simulink model "FuzzyLogicRobot_rev3"  (R2014a)
settings: Solver=ode45  SolverMode=SingleTasking  StartTime=0  StopTime=4.6  MaxStep=0.05  RelTol=1e-3  AbsTol=1e-6
libraries: simulink x3, fuzblock x1
CloseFcn:
  | AnimFigH = findobj(0,'Name', 'Tank Demo'); close(AnimFigH)
Description:
  | Control difuso de un robot móvil del tipo diferencial
settings Model: NumberOfSteps=10  LastModifiedBy=fravega
settings DataIOCC: LimitDataPoints=off  SignalLoggingSaveFormat=ModelDataLogs  SaveOutput=off  SaveTime=off
settings OptimizationCC: BlockReduction=off  BooleanDataType=off  ExpressionDepthLimit=2147483647  InitFltsAndDblsToZero=on
settings DebuggingCC: SaveWithParameterizedLinksMsg=none  UnderspecifiedInitializationDetection=Classic  SignalResolutionControl=TryResolveAllWithWarning  SolverPrmCheckMsg=none  MultiTaskDSMMsg=warning  MultiTaskCondExecSysMsg=none  FcnCallInpInsideContextMsg=UseLocalSettings  StateNameClashWarn=warning
settings HardwareCC: TargetLongLongMode=on  TargetEndianess=LittleEndian  TargetHWDeviceType=MATLAB Host  ProdEqTarget=off
settings RTWCC: GenerateMakefile=off  TemplateMakefile=grt_unix.tmf  IncludeERTFirstTime=on
settings GRTTargetCC: TargetFcnLib=ansi_tfl_tmw.mat  CombineOutputUpdateFcns=off  GRTInterface=on

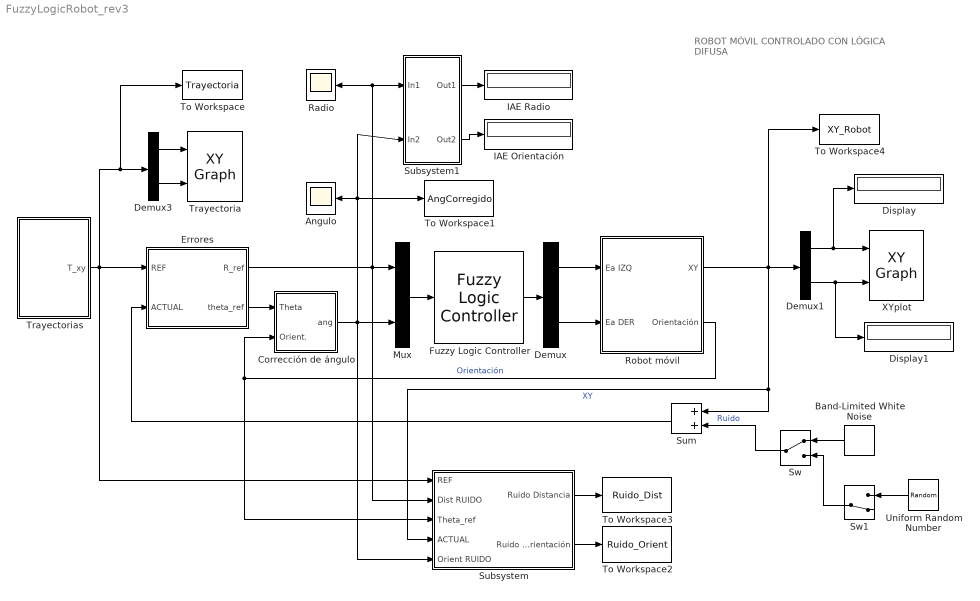
== system FuzzyLogicRobot_rev3 ==
  note: ROBOT MÓVIL CONTROLADO
      |  CON LÓGICA DIFUSA
  Angulo : Scope
      settings: TimeRange=5  YMin=-10  YMax=50  SaveName=ScopeData9
  Band-Limited White Noise : simulink/Sources/Band-Limited White Noise  Cov=[0.003]  Ts=0.1  seed=[23341]
  Corrección de ángulo : Subsystem
  Demux : Demux  Outputs=2
  Demux1 : Demux  Outputs=2
  Demux3 : Demux  Outputs=2
  Display : Display
  Display1 : Display
  Errores : Subsystem
  Fuzzy Logic Controller : fuzblock/Fuzzy Logic  Controller  fis='MRFL_rev33.fis'
  "IAE Orientación " : Display
  IAE Radio : Display
  Mux : Mux  Inputs=2
  Radio : Scope
      settings: TimeRange=5  YMin=0  SaveName=ScopeData10
  Robot móvil : Subsystem
      mask help:
      | Robot móvil del tipo Diferencial
      |
      | Entradas: Tensión de armadura de los motores de DC
      | Salidas: Posición en el plano (XY) y orientación
      mask Display: image('DDR.jpg')
  Subsystem : Subsystem
  Subsystem1 : Subsystem
  Sum : Sum
  Sw : ManualSwitch
  Sw1 : ManualSwitch  CurrentSetting=0
  To Workspace : ToWorkspace  VariableName=Trayectoria  SaveFormat=Timeseries  SampleTime=-1
  To Workspace1 : ToWorkspace  VariableName=AngCorregido  SaveFormat=Timeseries  SampleTime=-1
  To Workspace2 : ToWorkspace  VariableName=Ruido_Orient  SaveFormat=Timeseries  SampleTime=-1
  To Workspace3 : ToWorkspace  VariableName=Ruido_Dist  SaveFormat=Timeseries  SampleTime=-1
  To Workspace4 : ToWorkspace  VariableName=XY_Robot  SaveFormat=Timeseries  SampleTime=-1
  "Trayectoria " : simulink/Sinks/XY Graph  xmin=-4  xmax=4  ymin=-4  ymax=4  st=-1
  Trayectorias : Subsystem
  Uniform Random Number : UniformRandomNumber  SampleTime=0.1
  XYplot : simulink/Sinks/XY Graph  xmin=-4  xmax=4  ymin=-4  ymax=4  st=-1
  wires:
  Mux/1 -> Fuzzy Logic Controller/1
  Errores/2(theta_ref) -> Corrección de ángulo/1(Theta)
  Corrección de ángulo/1(ang) -> Angulo/1, To Workspace1/1, Subsystem1/2(In2), Subsystem/5(Orient RUIDO), Mux/2
  Trayectorias/1(T_xy) -> Subsystem/1(REF), Errores/1(REF), To Workspace/1, Demux3/1
  Robot móvil/1(XY) -> To Workspace4/1, Demux1/1, Sum/1, Subsystem/4(ACTUAL)  "XY"
  Errores/1(R_ref) -> Radio/1, Subsystem1/1(In1), Subsystem/2(Dist RUIDO), Mux/1
  Fuzzy Logic Controller/1 -> Demux/1
  Band-Limited White Noise/1 -> Sw/1
  Sw/1 -> Sum/2  "Ruido"
  Robot móvil/2(Orientación) -> Corrección de ángulo/2(Orient.), Subsystem/3(Theta_ref)  "Orientación"
  Sw1/1 -> Sw/2
  Uniform Random Number/1 -> Sw1/1
  Demux3/1 -> "Trayectoria "/1
  Demux3/2 -> "Trayectoria "/2
  Sum/1 -> Errores/2(ACTUAL)
  Demux/2 -> Robot móvil/2(Ea DER)
  Demux/1 -> Robot móvil/1(Ea IZQ)
  Demux1/1 -> XYplot/1, Display/1
  Demux1/2 -> Display1/1, XYplot/2
  Subsystem1/1(Out1) -> IAE Radio/1
  Subsystem1/2(Out2) -> "IAE Orientación "/1
  Subsystem/2(Ruido Orientación) -> To Workspace2/1
  Subsystem/1(Ruido Distancia) -> To Workspace3/1

== system FuzzyLogicRobot_rev3/Corrección de ángulo ==
  Theta : Inport
  Orient. : Inport  Port=2
  Corrección -180° a 180° : MATLABFcn  MATLABFcn=mod(u+180, 360) - 180
  Corregido : Scope
      settings: SaveName=ScopeData7
  Dif Ang : Scope
      settings: SaveName=ScopeData4
  Orientación : Scope
      settings: TimeRange=0.4  YMin=-45  YMax=-38
  Resta : Sum  Inputs=+-
  ang : Outport
  wires:
  Theta/1 -> Resta/1
  Corrección -180° a 180°/1 -> Corregido/1, ang/1
  Orient./1 -> Orientación/1, Resta/2
  Resta/1 -> Dif Ang/1, Corrección -180° a 180°/1

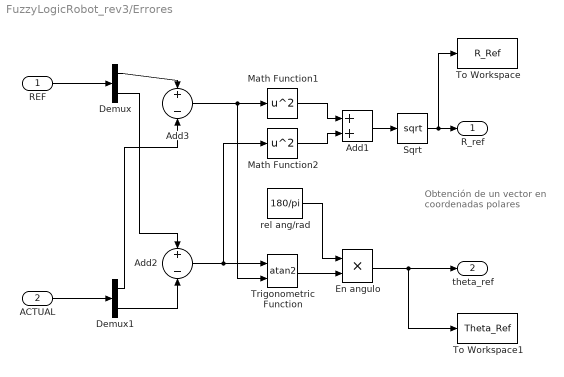
== system FuzzyLogicRobot_rev3/Errores ==
  note: Obtención de un vector
      | en coordenadas polares
  REF : Inport
  ACTUAL : Inport  Port=2
  Add1 : Sum
  Add2 : Sum  Inputs=+-
  Add3 : Sum  Inputs=+-
  Demux : Demux  Outputs=2
  Demux1 : Demux  Outputs=2
  En angulo : Product
  Math Function1 : Math  Operator=square  SaturateOnIntegerOverflow=on
  Math Function2 : Math  Operator=square  SaturateOnIntegerOverflow=on
  Sqrt : Sqrt  SaturateOnIntegerOverflow=on
  To Workspace : ToWorkspace  VariableName=R_Ref  SaveFormat=Timeseries  SampleTime=-1
  To Workspace1 : ToWorkspace  VariableName=Theta_Ref  SaveFormat=Timeseries  SampleTime=-1
  Trigonometric Function : Trigonometry  Operator=atan2
  rel ang/rad : Constant  Value=180/pi
  R_ref : Outport
  theta_ref : Outport  Port=2
  wires:
  Demux1/1 -> Add3/2
  Demux/2 -> Add2/1
  Demux1/2 -> Add2/2
  Demux/1 -> Add3/1
  Add1/1 -> Sqrt/1
  Math Function2/1 -> Add1/2
  Math Function1/1 -> Add1/1
  Add3/1 -> Trigonometric Function/2, Math Function1/1
  Add2/1 -> Math Function2/1, Trigonometric Function/1
  rel ang/rad/1 -> En angulo/1
  Trigonometric Function/1 -> En angulo/2
  En angulo/1 -> To Workspace1/1, theta_ref/1
  REF/1 -> Demux/1
  ACTUAL/1 -> Demux1/1
  Sqrt/1 -> To Workspace/1, R_ref/1

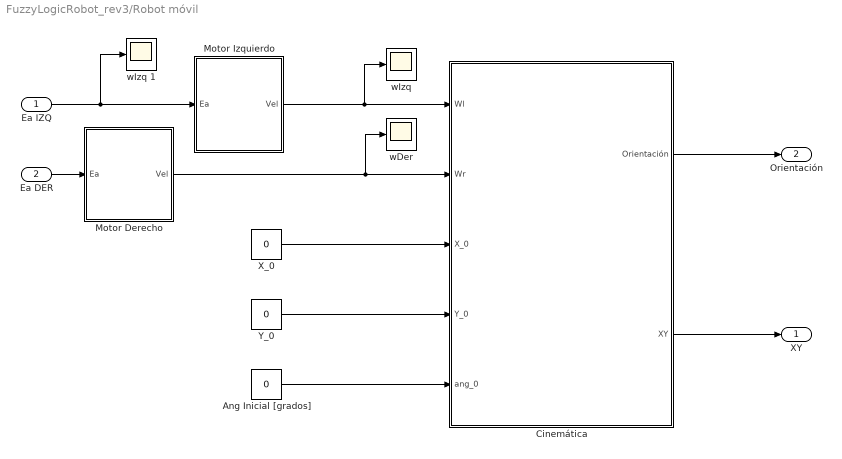
== system FuzzyLogicRobot_rev3/Robot móvil ==
  Ea IZQ : Inport
  Ea DER : Inport  Port=2
  Ang Inicial [grados] : Constant  Value=0
  Cinemática : Subsystem  Description=Cinemática directa del robot diferencial
  Motor Derecho : Subsystem
      mask Display: image('Motor.jpg')
  Motor Izquierdo : Subsystem
      mask Display: image('Motor.jpg')
  "X_0 " : Constant  Value=0
  Y_0 : Constant  Value=0
  wDer : Scope
      settings: TimeRange=20  YMin=0.194054  YMax=0.21448  SaveName=ScopeData3
  "wIzq " : Scope
      settings: TimeRange=20  YMin=0.194054  YMax=0.21448  SaveName=ScopeData2
  wIzq 1 : Scope
      settings: TimeRange=20  YMin=0  YMax=3.25  SaveName=ScopeData8
  XY : Outport
  Orientación : Outport  Port=2
  wires:
  Cinemática/2(XY) -> XY/1
  Cinemática/1(Orientación) -> Orientación/1
  "X_0 "/1 -> Cinemática/3(X_0)
  Y_0/1 -> Cinemática/4(Y_0)
  Ang Inicial [grados]/1 -> Cinemática/5(ang_0)
  Motor Izquierdo/1(Vel) -> "wIzq "/1, Cinemática/1(Wl)
  Ea IZQ/1 -> wIzq 1/1, Motor Izquierdo/1(Ea)
  Ea DER/1 -> Motor Derecho/1(Ea)
  Motor Derecho/1(Vel) -> wDer/1, Cinemática/2(Wr)

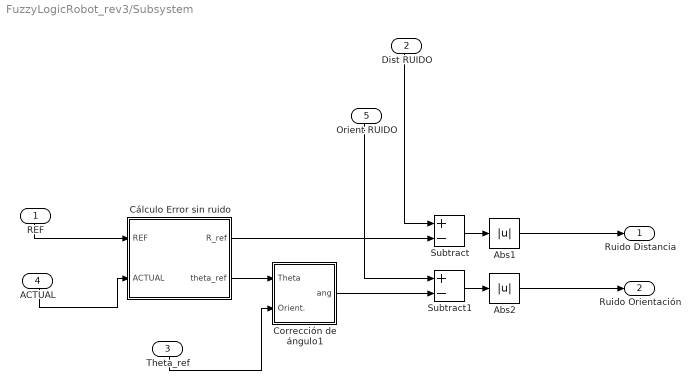
== system FuzzyLogicRobot_rev3/Subsystem ==
  REF : Inport
  Dist RUIDO : Inport  Port=2
  Theta_ref : Inport  Port=3
  ACTUAL : Inport  Port=4
  Orient RUIDO : Inport  Port=5
  Abs1 : Abs
  Abs2 : Abs
  Corrección de ángulo1 : Subsystem
  Cálculo Error sin ruido : Subsystem
  Subtract : Sum  Inputs=+-
  Subtract1 : Sum  Inputs=+-
  Ruido Distancia : Outport
  Ruido Orientación : Outport  Port=2
  wires:
  Orient RUIDO/1 -> Subtract1/1
  Cálculo Error sin ruido/2(theta_ref) -> Corrección de ángulo1/1(Theta)
  Abs2/1 -> Ruido Orientación/1
  Theta_ref/1 -> Corrección de ángulo1/2(Orient.)
  Dist RUIDO/1 -> Subtract/1
  REF/1 -> Cálculo Error sin ruido/1(REF)
  Cálculo Error sin ruido/1(R_ref) -> Subtract/2
  Subtract/1 -> Abs1/1
  Abs1/1 -> Ruido Distancia/1
  Corrección de ángulo1/1(ang) -> Subtract1/2
  ACTUAL/1 -> Cálculo Error sin ruido/2(ACTUAL)
  Subtract1/1 -> Abs2/1

== system FuzzyLogicRobot_rev3/Subsystem1 ==
  In1 : Inport
  In2 : Inport  Port=2
  Abs : Abs
  Integrator : Integrator
  Integrator1 : Integrator
  Out1 : Outport
  Out2 : Outport  Port=2
  wires:
  Integrator1/1 -> Out2/1
  Abs/1 -> Integrator1/1
  Integrator/1 -> Out1/1
  In2/1 -> Abs/1
  In1/1 -> Integrator/1

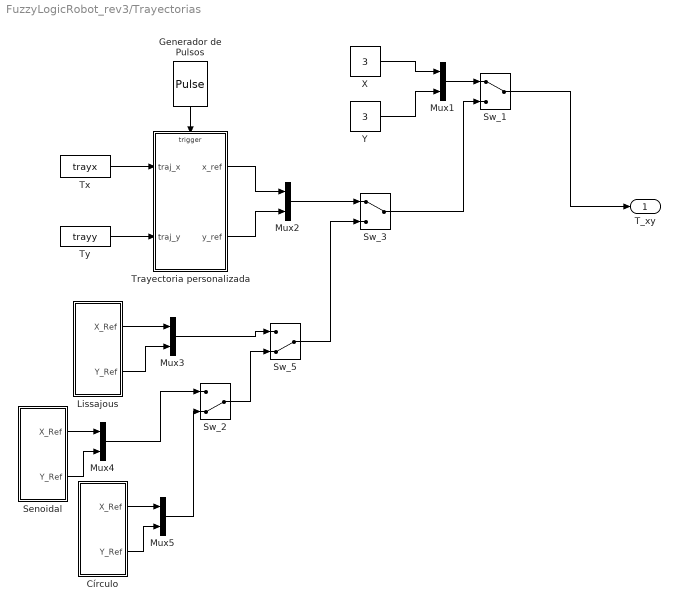
== system FuzzyLogicRobot_rev3/Trayectorias ==
  Círculo : Subsystem  AncestorBlock=roblocks/Trajectory/Circle  mask{freq=0.01}
      mask prompts: freq "Frequencia (rev/s)"
      mask help:
      | Genera una curva de Lissajous.
      | Para más info: http://es.wikipedia.org/wiki/Curva_de_Lissajous
  "Generador de Pulsos  " : DiscretePulseGenerator  PulseType=Time based  Period=1  PulseWidth=50
  Lissajous : Subsystem  AncestorBlock=roblocks/Trajectory/Circle  mask{freq=0.01}
      mask prompts: freq "Frequencia (rev/s)"
      mask help:
      | Genera una curva de Lissajous.
      | Para más info: http://es.wikipedia.org/wiki/Curva_de_Lissajous
  Mux{1..5} (5 alike) : Mux  Inputs=2
  Senoidal : Subsystem  AncestorBlock=roblocks/Trajectory/Circle  mask{freq=0.1}
      mask prompts: freq "Frequencia (rev/s)"
      mask help:
      | Genera una curva de Lissajous.
      | Para más info: http://es.wikipedia.org/wiki/Curva_de_Lissajous
  Sw_1 : ManualSwitch
  Sw_2 : ManualSwitch  CurrentSetting=0
  Sw_3 : ManualSwitch
  Sw_5 : ManualSwitch  CurrentSetting=0
  Trayectoria personalizada : Subsystem
  Tx : FromWorkspace  VariableName=trayx  SampleTime=0
  Ty : FromWorkspace  VariableName=trayy  SampleTime=0
  X : Constant  Value=3
  Y : Constant  Value=3
  T_xy : Outport
  wires:
  "Generador de Pulsos  "/1 -> Trayectoria personalizada/Trigger
  Tx/1 -> Trayectoria personalizada/1(traj_x)
  Ty/1 -> Trayectoria personalizada/2(traj_y)
  X/1 -> Mux1/1
  Y/1 -> Mux1/2
  Trayectoria personalizada/2(y_ref) -> Mux2/2
  Trayectoria personalizada/1(x_ref) -> Mux2/1
  Lissajous/1(X_Ref) -> Mux3/1
  Lissajous/2(Y_Ref) -> Mux3/2
  Senoidal/1(X_Ref) -> Mux4/1
  Senoidal/2(Y_Ref) -> Mux4/2
  Mux3/1 -> Sw_5/1
  Mux1/1 -> Sw_1/1
  Sw_1/1 -> T_xy/1
  Mux2/1 -> Sw_3/1
  Sw_5/1 -> Sw_3/2
  Sw_3/1 -> Sw_1/2
  Círculo/1(X_Ref) -> Mux5/1
  Círculo/2(Y_Ref) -> Mux5/2
  Mux5/1 -> Sw_2/2
  Sw_2/1 -> Sw_5/2
  Mux4/1 -> Sw_2/1

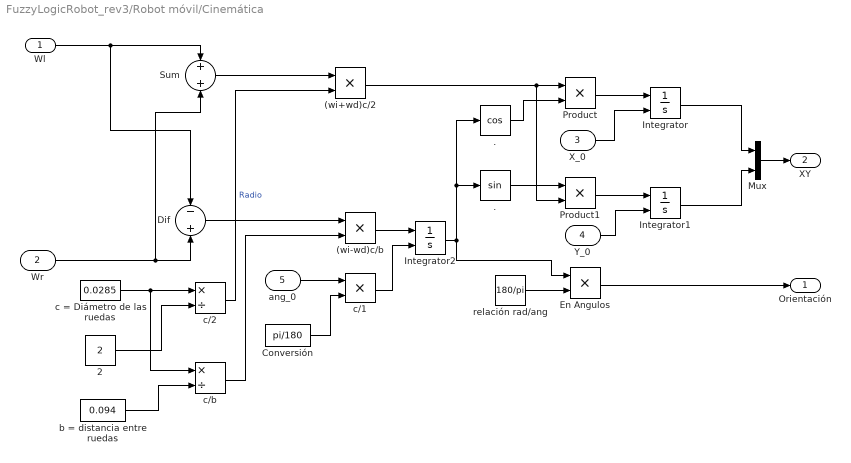
== system FuzzyLogicRobot_rev3/Robot móvil/Cinemática ==
  Wl : Inport
  Wr : Inport  Port=2
  X_0 : Inport  Port=3
  Y_0 : Inport  Port=4
  ang_0 : Inport  Port=5
  (wi+wd)c/2 : Product  RndMeth=Zero
  (wi-wd)c/b : Product  RndMeth=Zero
  . : Trigonometry
  ". " : Trigonometry  Operator=cos
  2 : Constant  Value=2
  Conversión : Constant  Value=pi/180
  Dif : Sum  Inputs=-+
  En Angulos : Product  RndMeth=Zero
  Integrator : Integrator  InitialConditionSource=external
  Integrator1 : Integrator  InitialConditionSource=external
  Integrator2 : Integrator  InitialConditionSource=external
  Mux : Mux  Inputs=2
  Product : Product  RndMeth=Zero
  Product1 : Product  RndMeth=Zero
  Sum : Sum
  b = distancia entre ruedas : Constant  Value=0.094
  c = Diámetro de las ruedas : Constant  Value=0.0285
  c/1 : Product  Inputs=**
  c/2 : Product  Inputs=*/
  c/b : Product  Inputs=*/
  "relación rad/ang " : Constant  Value=180/pi
  Orientación : Outport
  XY : Outport  Port=2
  wires:
  Product/1 -> Integrator/1
  Product1/1 -> Integrator1/1
  (wi+wd)c/2/1 -> Product1/2, Product/1
  (wi-wd)c/b/1 -> Integrator2/1
  Dif/1 -> (wi-wd)c/b/1
  Sum/1 -> (wi+wd)c/2/1
  Wr/1 -> Sum/2, Dif/2
  Wl/1 -> Dif/1, Sum/1
  Integrator/1 -> Mux/1
  Integrator1/1 -> Mux/2
  ". "/1 -> Product/2
  ./1 -> Product1/1
  c = Diámetro de las ruedas/1 -> c/2/1, c/b/1
  b = distancia entre ruedas/1 -> c/b/2
  2/1 -> c/2/2
  c/2/1 -> (wi+wd)c/2/2  "Radio"
  c/b/1 -> (wi-wd)c/b/2
  X_0/1 -> Integrator/2
  Y_0/1 -> Integrator1/2
  ang_0/1 -> c/1/1
  Conversión/1 -> c/1/2
  Integrator2/1 -> En Angulos/1, ". "/1, ./1
  c/1/1 -> Integrator2/2
  "relación rad/ang "/1 -> En Angulos/2
  Mux/1 -> XY/1
  En Angulos/1 -> Orientación/1

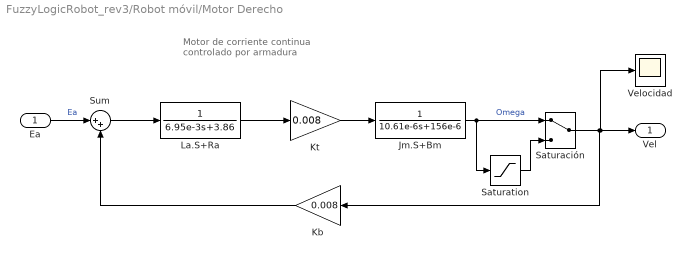
== system FuzzyLogicRobot_rev3/Robot móvil/Motor Derecho ==
  note: Motor de corriente continua
      | controlado por armadura
  Ea : Inport
  Jm.S+Bm : TransferFcn  Denominator=[10.61e-6 156e-6]
  Kb : Gain  Gain=0.008
  Kt : Gain  Gain=0.008
  La.S+Ra : TransferFcn  Denominator=[6.95e-3 3.86]
  Saturación : ManualSwitch
  Saturation : Saturate  UpperLimit=30  LowerLimit=-30
  Sum : Sum  Inputs=|++
  Velocidad : Scope
  Vel : Outport
  wires:
  La.S+Ra/1 -> Kt/1
  Kb/1 -> Sum/2
  Kt/1 -> Jm.S+Bm/1
  Sum/1 -> La.S+Ra/1
  Ea/1 -> Sum/1  "Ea"
  Jm.S+Bm/1 -> Saturación/1, Saturation/1  "Omega"
  Saturation/1 -> Saturación/2
  Saturación/1 -> Kb/1, Velocidad/1, Vel/1

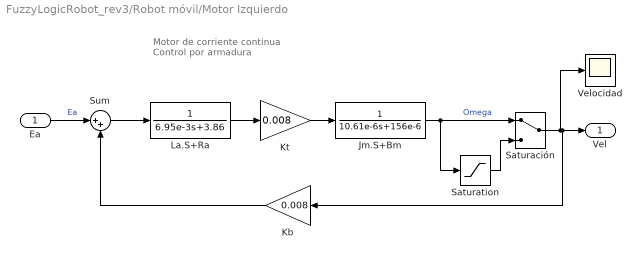
== system FuzzyLogicRobot_rev3/Robot móvil/Motor Izquierdo ==
  note: Motor de corriente continua
      | Control por armadura
  Ea : Inport
  Jm.S+Bm : TransferFcn  Denominator=[10.61e-6 156e-6]
  Kb : Gain  Gain=0.008
  Kt : Gain  Gain=0.008
  La.S+Ra : TransferFcn  Denominator=[ 6.95e-3 3.86]
  Saturación : ManualSwitch
  Saturation : Saturate  UpperLimit=30  LowerLimit=-30
  Sum : Sum  Inputs=|++
  Velocidad : Scope
  Vel : Outport
  wires:
  La.S+Ra/1 -> Kt/1
  Kb/1 -> Sum/2
  Kt/1 -> Jm.S+Bm/1
  Sum/1 -> La.S+Ra/1
  Ea/1 -> Sum/1  "Ea"
  Jm.S+Bm/1 -> Saturation/1, Saturación/1  "Omega"
  Saturación/1 -> Vel/1, Kb/1, Velocidad/1
  Saturation/1 -> Saturación/2

== system FuzzyLogicRobot_rev3/Subsystem/Corrección de ángulo1 ==
  Theta : Inport
  Orient. : Inport  Port=2
  Corrección -180° a 180° : MATLABFcn  MATLABFcn=mod(u+180, 360) - 180
  Corregido : Scope
      settings: SaveName=ScopeData7
  Dif Ang : Scope
      settings: SaveName=ScopeData4
  Orientación : Scope
      settings: TimeRange=0.4  YMin=-45  YMax=-38
  Resta : Sum  Inputs=+-
  ang : Outport
  wires:
  Resta/1 -> Corrección -180° a 180°/1, Dif Ang/1
  Orient./1 -> Resta/2, Orientación/1
  Corrección -180° a 180°/1 -> ang/1, Corregido/1
  Theta/1 -> Resta/1

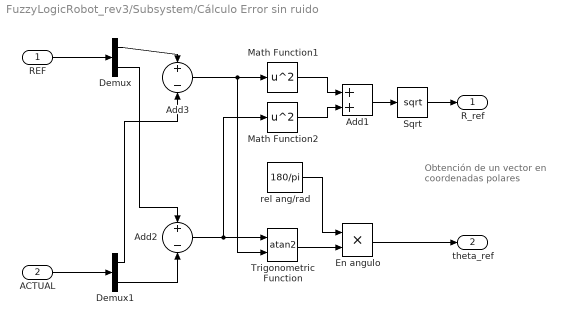
== system FuzzyLogicRobot_rev3/Subsystem/Cálculo Error sin ruido ==
  note: Obtención de un vector
      | en coordenadas polares
  REF : Inport
  ACTUAL : Inport  Port=2
  Add1 : Sum
  Add2 : Sum  Inputs=+-
  Add3 : Sum  Inputs=+-
  Demux : Demux  Outputs=2
  Demux1 : Demux  Outputs=2
  En angulo : Product
  Math Function1 : Math  Operator=square  SaturateOnIntegerOverflow=on
  Math Function2 : Math  Operator=square  SaturateOnIntegerOverflow=on
  Sqrt : Sqrt  SaturateOnIntegerOverflow=on
  Trigonometric Function : Trigonometry  Operator=atan2
  rel ang/rad : Constant  Value=180/pi
  R_ref : Outport
  theta_ref : Outport  Port=2
  wires:
  Sqrt/1 -> R_ref/1
  ACTUAL/1 -> Demux1/1
  REF/1 -> Demux/1
  En angulo/1 -> theta_ref/1
  Trigonometric Function/1 -> En angulo/2
  rel ang/rad/1 -> En angulo/1
  Add2/1 -> Trigonometric Function/1, Math Function2/1
  Add3/1 -> Math Function1/1, Trigonometric Function/2
  Math Function1/1 -> Add1/1
  Math Function2/1 -> Add1/2
  Add1/1 -> Sqrt/1
  Demux/1 -> Add3/1
  Demux1/2 -> Add2/2
  Demux/2 -> Add2/1
  Demux1/1 -> Add3/2

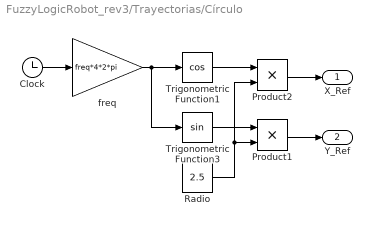
== system FuzzyLogicRobot_rev3/Trayectorias/Círculo ==
  Clock : Clock
  Product1 : Product
  Product2 : Product
  Radio : Constant  Value=2.5
  Trigonometric Function1 : Trigonometry  Operator=cos
  Trigonometric Function3 : Trigonometry
  freq : Gain  Gain=freq*4*2*pi
  X_Ref : Outport
  Y_Ref : Outport  Port=2
  wires:
  Clock/1 -> freq/1
  Product1/1 -> Y_Ref/1
  freq/1 -> Trigonometric Function3/1, Trigonometric Function1/1
  Trigonometric Function1/1 -> Product2/1
  Trigonometric Function3/1 -> Product1/1
  Radio/1 -> Product1/2, Product2/2
  Product2/1 -> X_Ref/1

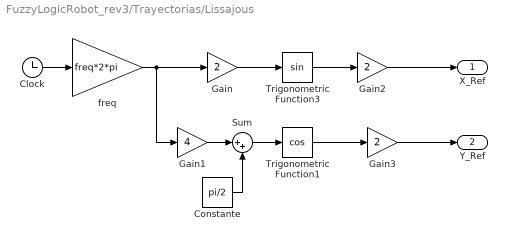
== system FuzzyLogicRobot_rev3/Trayectorias/Lissajous ==
  Clock : Clock
  Constante : Constant  Value=pi/2
  Gain : Gain  Gain=2
  Gain1 : Gain  Gain=4
  Gain2 : Gain  Gain=2
  Gain3 : Gain  Gain=2
  Sum : Sum  Inputs=|++
  Trigonometric Function1 : Trigonometry  Operator=cos
  Trigonometric Function3 : Trigonometry
  freq : Gain  Gain=freq*2*pi
  X_Ref : Outport
  Y_Ref : Outport  Port=2
  wires:
  Clock/1 -> freq/1
  freq/1 -> Gain1/1, Gain/1
  Gain/1 -> Trigonometric Function3/1
  Gain1/1 -> Sum/1
  Sum/1 -> Trigonometric Function1/1
  Constante/1 -> Sum/2
  Trigonometric Function3/1 -> Gain2/1
  Gain2/1 -> X_Ref/1
  Trigonometric Function1/1 -> Gain3/1
  Gain3/1 -> Y_Ref/1

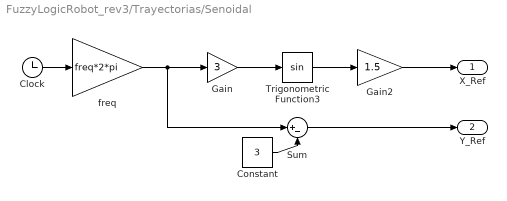
== system FuzzyLogicRobot_rev3/Trayectorias/Senoidal ==
  Clock : Clock
  Constant : Constant  Value=3
  Gain : Gain  Gain=3
  Gain2 : Gain  Gain=1.5
  Sum : Sum  Inputs=|+-
  Trigonometric Function3 : Trigonometry
  freq : Gain  Gain=freq*2*pi
  X_Ref : Outport
  Y_Ref : Outport  Port=2
  wires:
  Clock/1 -> freq/1
  Gain/1 -> Trigonometric Function3/1
  Trigonometric Function3/1 -> Gain2/1
  Gain2/1 -> X_Ref/1
  freq/1 -> Sum/1, Gain/1
  Constant/1 -> Sum/2
  Sum/1 -> Y_Ref/1

== system FuzzyLogicRobot_rev3/Trayectorias/Trayectoria personalizada ==
  note: Cada disparo agarra un nuevo punto
  traj_x : Inport
  traj_y : Inport  Port=2
  Trigger : TriggerPort
  Discretización : MATLAB Function  TreatAsAtomicUnit=on
  x_ref : Outport
  y_ref : Outport  Port=2
  wires:
  Discretización/1(x) -> x_ref/1
  traj_x/1 -> Discretización/1(tx)
  Discretización/2(y) -> y_ref/1
  traj_y/1 -> Discretización/2(ty)

== matlab function FuzzyLogicRobot_rev3/Trayectorias/Trayectoria personalizada/Discretización ==
  data: x output; tx input; ty input; y output
function [x,y] = fcn(tx,ty)
% Input:  (tx,ty): Trayectorias
% Output: (x,y)  : Valores discretizados

persistent i;

if isempty(i) 
    i = 1;
end
    x = tx(i);          % Toma el valor i-ésimo del vector tx[].
    y = ty(i);

    if i < length(tx)   % Verifica que no se recorrido 
        i = i+1;        % todo el vector de trayectorias
    end
